simulink model "TrafficLight"  (R2024b)
settings: Solver=VariableStepAuto  StartTime=0.0  StopTime=100  RelTol=1e-3
libraries: simulink x1
settings Model: Creator=Matthew  LastModifiedBy=Matthew

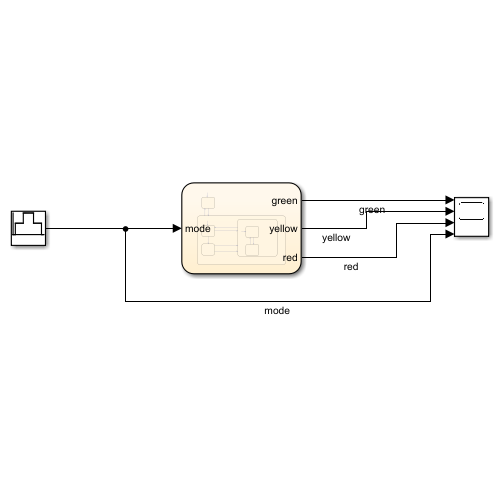
[thumbnail: Simulink's stored preview of the top-level diagram]
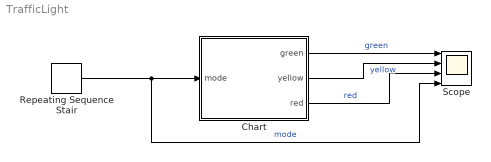
== system TrafficLight ==
  Chart : Stateflow chart  TreatAsAtomicUnit=on
  Repeating Sequence Stair : simulink/Sources/Repeating Sequence Stair  OutValues=[0 0 0 0 0 0 0 0 1 1 1 1 1 1 1 1 1 1 1 1 1 1 1 1 1 1 1 2 2 2 2 2 2 2 2 2 2 2 2 2 2 2 2 2 2 2 2 2 2 2 2 1 1 1 1 1 1 1 1 1 1 1 1 1 1 1 1 1 1 1 0 0 0 0 0 0 0].'  tsamp=1  OutMin=[]  OutMax=[]  OutDataTypeStr=double  OutputDataTypeScalingMode=double  OutDataType=fixdt(0,8)  ConRadixGroup=Best Precision: Vector-wise  OutScaling=2^-12
  Scope : Scope  NumInputPorts=4
  wires:
  Chart/1(green) -> Scope/1  "green"
  Chart/2(yellow) -> Scope/2  "yellow"
  Chart/3(red) -> Scope/3  "red"
  Repeating Sequence Stair/1 -> Scope/4, Chart/1(mode)  "mode"

== stateflow chart TrafficLight/Chart ==
  state Off
    entry:
    green=0;
    red=0;
    yellow=0;
  state Active
    state Red
      state On
        entry:
        green=0;
        red=1;
        yellow=0;
      state Off
        entry:
        green=0;
        red=0;
        yellow=0;
      (default) -> On
      Active.Red.Off -> On : after(1,sec)
      On -> Active.Red.Off : after(1,sec) [mode==2]
    state Green
      entry:
      green=1;
      red=0;
      yellow=0;
    state Yellow
      entry:
      green=0;
      red=0;
      yellow=1;
    (default) -> Green
    Red -> Green : after(3,sec)[mode==1]
    Green -> Red [order 2] : [mode==2]
    Green -> Yellow [order 1] : after(3,sec)
    Yellow -> Red [order 1] : after(1,sec)
    Yellow -> Red [order 2] : [mode==2]
  (default) -> Off
  Active -> Off : [mode==0]
  Off -> Active : [mode~=0]
  data: green output; yellow output; red output; mode input
